simulink model "exp5_9"  (Simulink 3.00)
settings: Solver=FixedStepDiscrete  SolverMode=SingleTasking  StartTime=0.0  StopTime=10.0  RelTol=1e-3  AbsTol=1e-6
settings Model: TimeSaveName=t  OutputSaveName=y  RTWTemplateMakefile=grt_vc.tmf

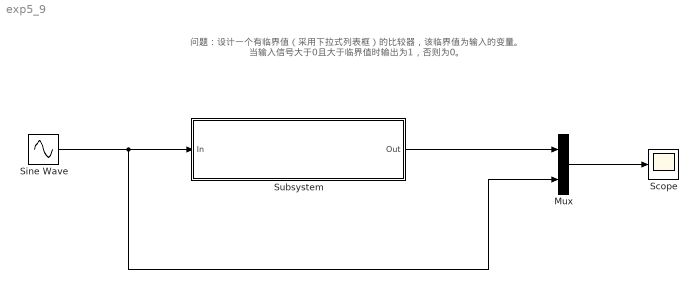
== system exp5_9 ==
  note: 问题：设计一个有临界值（采用下拉式列表框）的比较器，该临界值为输入的变量。
      | 当输入信号大于0且大于临界值时输出为1，否则为0。
  Mux : Mux  Inputs=2
  Scope : Scope
      settings: TickLabels=on  TimeRange=10  YMin=-5  YMax=5  SaveToWorkspace=off  SaveName=ScopeData  DataFormat=Matrix
  Sine Wave : Sin  Amplitude=5  Frequency=1  Phase=0  SampleTime=0
  Subsystem : Subsystem  mask(comparater){th=0.3}
      mask prompts: th "threshold"
      mask StyleString: popup(0.1|0.2|0.3)
      mask Display: disp('The Comparater')
  wires:
  Subsystem/1(Out) -> Mux/1
  Mux/1 -> Scope/1
  Sine Wave/1 -> Subsystem/1(In), Mux/2

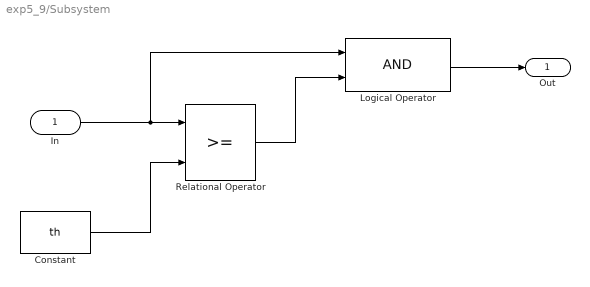
== system exp5_9/Subsystem ==
  In : Inport  Port=1  PortWidth=-1  SampleTime=-1  DataType=auto
      settings: SignalType=auto
  Constant : Constant  Value=th
  Logical Operator : Logic  Operator=AND  Inputs=2
  Relational Operator : RelationalOperator  Operator=>=
  Out : Outport  Port=1  InitialOutput=0
  wires:
  Logical Operator/1 -> Out/1
  In/1 -> Logical Operator/1, Relational Operator/1
  Constant/1 -> Relational Operator/2
  Relational Operator/1 -> Logical Operator/2
